simulink model "modelo_cinematico"  (Simulink 7.5)
settings: Solver=ode45  StartTime=0.0  StopTime=10.0  RelTol=1e-3
libraries: simulink x1
settings Model: Creator=ARTURO  LastModifiedBy=ARTURO

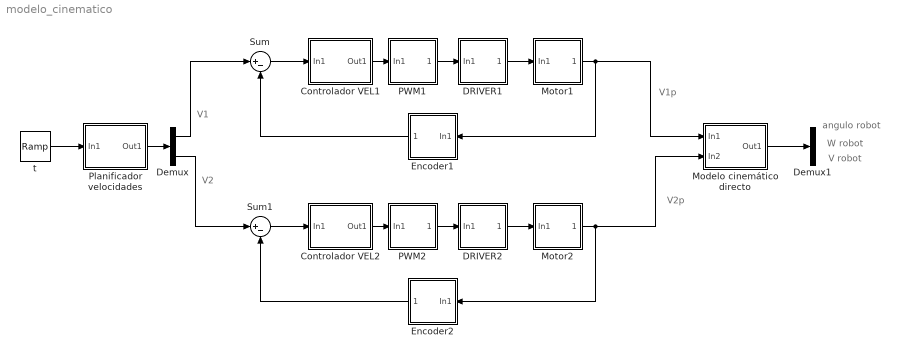
== system modelo_cinematico ==
  note: V1
  note: V2
  note: V1p
  note: V2p
  note: W robot
  note: V robot
  note: angulo robot
  Controlador VEL1 : Subsystem
  Controlador VEL2 : Subsystem
  DRIVER1 : Subsystem
  DRIVER2 : Subsystem
  Demux : Demux  Outputs=2
  Demux1 : Demux  Outputs=3
  Encoder1 : Subsystem
  Encoder2 : Subsystem
  Modelo cinemático directo : Subsystem
  Motor1 : Subsystem
  Motor2 : Subsystem
  PWM1 : Subsystem
  PWM2 : Subsystem
  Planificador velocidades : Subsystem
  Sum : Sum  Inputs=|+-  OutDataType=fixdt(1, 16)  OutScaling=2^0
  Sum1 : Sum  Inputs=|+-  OutDataType=fixdt(1, 16)  OutScaling=2^0
  t : simulink/Sources/Ramp  SystemSampleTime=-1  slope=1  start=0  X0=0
  wires:
  Sum/1 -> Controlador VEL1/1(In1)
  Controlador VEL1/1(Out1) -> PWM1/1(In1)
  PWM1/1(Out1) -> DRIVER1/1(In1)
  DRIVER1/1(Out1) -> Motor1/1(In1)
  Motor1/1(Out1) -> Encoder1/1(In1), Modelo cinemático directo/1(In1)
  Encoder1/1(Out1) -> Sum/2
  Demux/1 -> Sum/1
  Sum1/1 -> Controlador VEL2/1(In1)
  Controlador VEL2/1(Out1) -> PWM2/1(In1)
  PWM2/1(Out1) -> DRIVER2/1(In1)
  DRIVER2/1(Out1) -> Motor2/1(In1)
  Motor2/1(Out1) -> Encoder2/1(In1), Modelo cinemático directo/2(In2)
  Encoder2/1(Out1) -> Sum1/2
  Demux/2 -> Sum1/1
  Planificador velocidades/1(Out1) -> Demux/1
  t/1 -> Planificador velocidades/1(In1)
  Modelo cinemático directo/1(Out1) -> Demux1/1

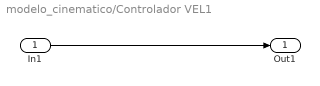
== system modelo_cinematico/Controlador VEL1 ==
  In1 : Inport  OutDataType=fixdt(1, 16)  OutScaling=2^0
  Out1 : Outport  OutDataType=fixdt(1, 16)  OutScaling=2^0
  wires:
  In1/1 -> Out1/1

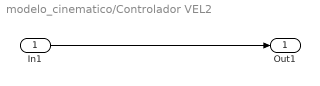
== system modelo_cinematico/Controlador VEL2 ==
  In1 : Inport  OutDataType=fixdt(1, 16)  OutScaling=2^0
  Out1 : Outport  OutDataType=fixdt(1, 16)  OutScaling=2^0
  wires:
  In1/1 -> Out1/1

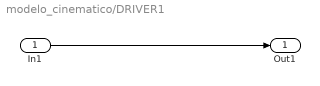
== system modelo_cinematico/DRIVER1 ==
  In1 : Inport  OutDataType=fixdt(1, 16)  OutScaling=2^0
  Out1 : Outport  OutDataType=fixdt(1, 16)  OutScaling=2^0
  wires:
  In1/1 -> Out1/1

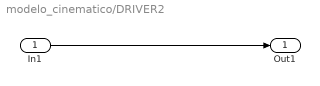
== system modelo_cinematico/DRIVER2 ==
  In1 : Inport  OutDataType=fixdt(1, 16)  OutScaling=2^0
  Out1 : Outport  OutDataType=fixdt(1, 16)  OutScaling=2^0
  wires:
  In1/1 -> Out1/1

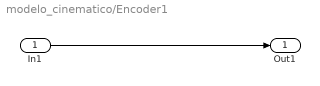
== system modelo_cinematico/Encoder1 ==
  In1 : Inport  OutDataType=fixdt(1, 16)  OutScaling=2^0
  Out1 : Outport  OutDataType=fixdt(1, 16)  OutScaling=2^0
  wires:
  In1/1 -> Out1/1

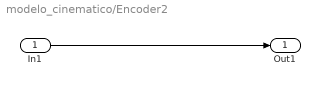
== system modelo_cinematico/Encoder2 ==
  In1 : Inport  OutDataType=fixdt(1, 16)  OutScaling=2^0
  Out1 : Outport  OutDataType=fixdt(1, 16)  OutScaling=2^0
  wires:
  In1/1 -> Out1/1

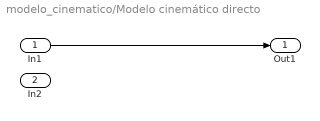
== system modelo_cinematico/Modelo cinemático directo ==
  In1 : Inport  OutDataType=fixdt(1, 16)  OutScaling=2^0
  In2 : Inport  Port=2  OutDataType=fixdt(1, 16)  OutScaling=2^0
  Out1 : Outport  OutDataType=fixdt(1, 16)  OutScaling=2^0
  wires:
  In1/1 -> Out1/1

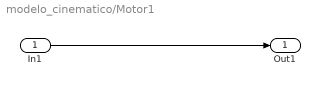
== system modelo_cinematico/Motor1 ==
  In1 : Inport  OutDataType=fixdt(1, 16)  OutScaling=2^0
  Out1 : Outport  OutDataType=fixdt(1, 16)  OutScaling=2^0
  wires:
  In1/1 -> Out1/1

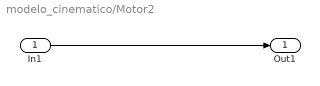
== system modelo_cinematico/Motor2 ==
  In1 : Inport  OutDataType=fixdt(1, 16)  OutScaling=2^0
  Out1 : Outport  OutDataType=fixdt(1, 16)  OutScaling=2^0
  wires:
  In1/1 -> Out1/1

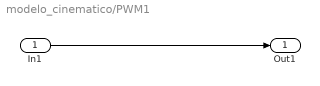
== system modelo_cinematico/PWM1 ==
  In1 : Inport  OutDataType=fixdt(1, 16)  OutScaling=2^0
  Out1 : Outport  OutDataType=fixdt(1, 16)  OutScaling=2^0
  wires:
  In1/1 -> Out1/1

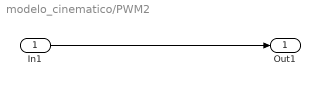
== system modelo_cinematico/PWM2 ==
  In1 : Inport  OutDataType=fixdt(1, 16)  OutScaling=2^0
  Out1 : Outport  OutDataType=fixdt(1, 16)  OutScaling=2^0
  wires:
  In1/1 -> Out1/1

== system modelo_cinematico/Planificador velocidades ==
  In1 : Inport  OutDataType=fixdt(1, 16)  OutScaling=2^0
  Out1 : Outport  OutDataType=fixdt(1, 16)  OutScaling=2^0
  wires:
  In1/1 -> Out1/1
